simulink model "TST_DReqSwt_DD"  (R2016b)
settings: Solver=FixedStepDiscrete  StartTime=0.0  StopTime=simTime  FixedStep=sampleTime  RelTol=1e-3
values from neighbouring files (symbols this model uses):
  testCase = 1    [initTST_DReqSwt_DD_001.m]
libraries: simulink x4, UnitTest_Lib x2
settings Model: Creator=xinchangran  LastModifiedBy=xinchangran
settings DebuggingCC: SignalRangeChecking=error

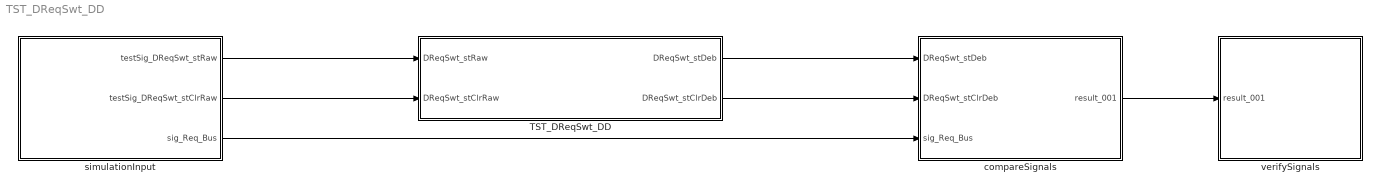
== system TST_DReqSwt_DD ==
  TST_DReqSwt_DD : Subsystem
  compareSignals : Subsystem
  simulationInput : Subsystem
  verifySignals : Subsystem
  wires:
  simulationInput/1(testSig_DReqSwt_stRaw) -> TST_DReqSwt_DD/1(DReqSwt_stRaw)
  simulationInput/2(testSig_DReqSwt_stClrRaw) -> TST_DReqSwt_DD/2(DReqSwt_stClrRaw)
  TST_DReqSwt_DD/1(DReqSwt_stDeb) -> compareSignals/1(DReqSwt_stDeb)
  TST_DReqSwt_DD/2(DReqSwt_stClrDeb) -> compareSignals/2(DReqSwt_stClrDeb)
  simulationInput/3(sig_Req_Bus) -> compareSignals/3(sig_Req_Bus)
  compareSignals/1(result_001) -> verifySignals/1(result_001)

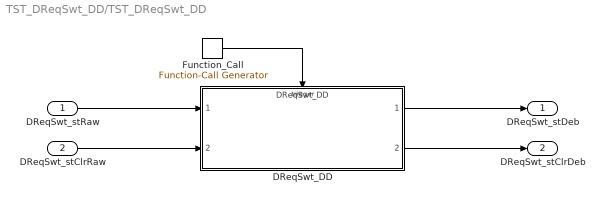
== system TST_DReqSwt_DD/TST_DReqSwt_DD ==
  DReqSwt_stRaw : Inport
  DReqSwt_stClrRaw : Inport  Port=2
  DReqSwt_DD : ModelReference  ModelNameDialog=DReqSwt_DD  SimulationMode=Normal  ModelReferenceVersion=1.17  TriggerPortName=function  TriggerPortTriggerType=function-call  TriggerPortStatesWhenEnabling=held
  Function_Call : simulink/Ports & Subsystems/Function-Call Generator  sample_time=sampleTime  numberOfIterations=1
  DReqSwt_stDeb : Outport
  DReqSwt_stClrDeb : Outport  Port=2
  wires:
  Function_Call/1 -> DReqSwt_DD/Trigger
  DReqSwt_stRaw/1 -> DReqSwt_DD/1
  DReqSwt_stClrRaw/1 -> DReqSwt_DD/2
  DReqSwt_DD/1 -> DReqSwt_stDeb/1
  DReqSwt_DD/2 -> DReqSwt_stClrDeb/1

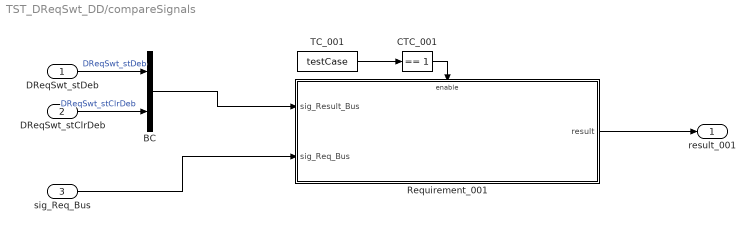
== system TST_DReqSwt_DD/compareSignals ==
  DReqSwt_stDeb : Inport
  DReqSwt_stClrDeb : Inport  Port=2
  sig_Req_Bus : Inport  Port=3
  BC : BusCreator  Inputs=2
  CTC_001 : simulink/Logic and Bit Operations/Compare To Constant  relop===  const=1  OutDataTypeStr=boolean
  Requirement_001 : Subsystem
  TC_001 : Constant  Value=testCase
  result_001 : Outport
  wires:
  DReqSwt_stDeb/1 -> BC/1  "DReqSwt_stDeb"
  DReqSwt_stClrDeb/1 -> BC/2  "DReqSwt_stClrDeb"
  TC_001/1 -> CTC_001/1
  CTC_001/1 -> Requirement_001/Enable
  sig_Req_Bus/1 -> Requirement_001/2(sig_Req_Bus)
  BC/1 -> Requirement_001/1(sig_Result_Bus)
  Requirement_001/1(result) -> result_001/1

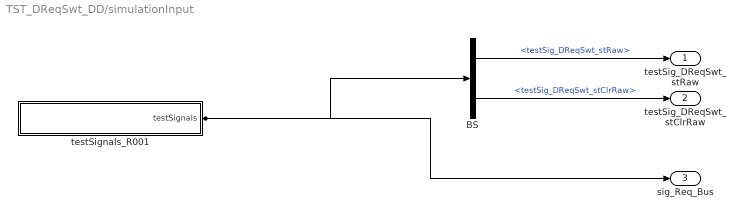
== system TST_DReqSwt_DD/simulationInput ==
  BS : BusSelector  OutputSignals=testSig_DReqSwt_stRaw,testSig_DReqSwt_stClrRaw
  testSignals_R001 : Subsystem
  testSig_DReqSwt_stRaw : Outport
  testSig_DReqSwt_stClrRaw : Outport  Port=2
  sig_Req_Bus : Outport  Port=3
  wires:
  BS/1 -> testSig_DReqSwt_stRaw/1  "<testSig_DReqSwt_stRaw>"
  BS/2 -> testSig_DReqSwt_stClrRaw/1  "<testSig_DReqSwt_stClrRaw>"
  testSignals_R001/1(testSignals) -> BS/1, sig_Req_Bus/1

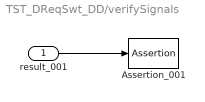
== system TST_DReqSwt_DD/verifySignals ==
  result_001 : Inport
  Assertion_001 : Assertion  Enabled=off
  wires:
  result_001/1 -> Assertion_001/1

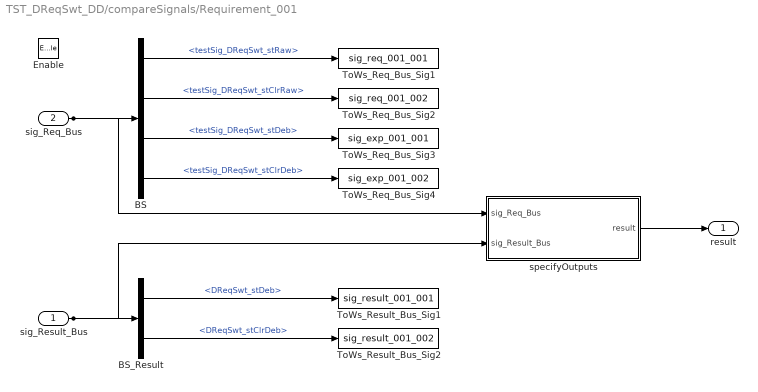
== system TST_DReqSwt_DD/compareSignals/Requirement_001 ==
  sig_Result_Bus : Inport
  sig_Req_Bus : Inport  Port=2
  Enable : EnablePort
  BS : BusSelector  OutputSignals=testSig_DReqSwt_stRaw,testSig_DReqSwt_stClrRaw,testSig_DReqSwt_stDeb,testSig_DReqSwt_stClrDeb
  BS_Result : BusSelector  OutputSignals=DReqSwt_stDeb,DReqSwt_stClrDeb
  ToWs_Req_Bus_Sig1 : ToWorkspace  VariableName=sig_req_001_001  SaveFormat=Structure With Time
  ToWs_Req_Bus_Sig2 : ToWorkspace  VariableName=sig_req_001_002  SaveFormat=Structure With Time
  ToWs_Req_Bus_Sig3 : ToWorkspace  VariableName=sig_exp_001_001  SaveFormat=Structure With Time
  ToWs_Req_Bus_Sig4 : ToWorkspace  VariableName=sig_exp_001_002  SaveFormat=Structure With Time
  ToWs_Result_Bus_Sig1 : ToWorkspace  VariableName=sig_result_001_001  SaveFormat=Structure With Time
  ToWs_Result_Bus_Sig2 : ToWorkspace  VariableName=sig_result_001_002  SaveFormat=Structure With Time
  specifyOutputs : Subsystem
  result : Outport
  wires:
  sig_Req_Bus/1 -> BS/1, specifyOutputs/1(sig_Req_Bus)
  BS/1 -> ToWs_Req_Bus_Sig1/1  "<testSig_DReqSwt_stRaw>"
  BS/2 -> ToWs_Req_Bus_Sig2/1  "<testSig_DReqSwt_stClrRaw>"
  BS/3 -> ToWs_Req_Bus_Sig3/1  "<testSig_DReqSwt_stDeb>"
  BS/4 -> ToWs_Req_Bus_Sig4/1  "<testSig_DReqSwt_stClrDeb>"
  sig_Result_Bus/1 -> BS_Result/1, specifyOutputs/2(sig_Result_Bus)
  BS_Result/1 -> ToWs_Result_Bus_Sig1/1  "<DReqSwt_stDeb>"
  BS_Result/2 -> ToWs_Result_Bus_Sig2/1  "<DReqSwt_stClrDeb>"
  specifyOutputs/1(result) -> result/1

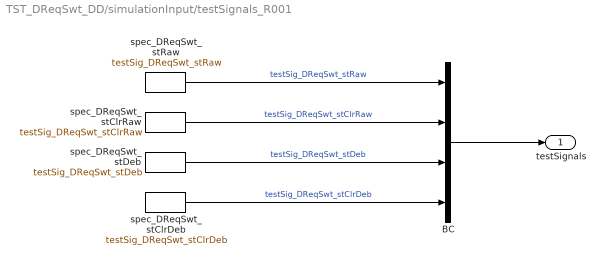
== system TST_DReqSwt_DD/simulationInput/testSignals_R001 ==
  BC : BusCreator  Inputs=4
  spec_DReqSwt_stClrDeb : FromWorkspace  VariableName=testSig_DReqSwt_stClrDeb  Interpolate=off  OutputAfterFinalValue=Holding final value
  spec_DReqSwt_stClrRaw : FromWorkspace  VariableName=testSig_DReqSwt_stClrRaw  Interpolate=off  OutputAfterFinalValue=Holding final value
  spec_DReqSwt_stDeb : FromWorkspace  VariableName=testSig_DReqSwt_stDeb  Interpolate=off  OutputAfterFinalValue=Holding final value
  spec_DReqSwt_stRaw : FromWorkspace  VariableName=testSig_DReqSwt_stRaw  Interpolate=off  OutputAfterFinalValue=Holding final value
  testSignals : Outport
  wires:
  BC/1 -> testSignals/1
  spec_DReqSwt_stRaw/1 -> BC/1  "testSig_DReqSwt_stRaw"
  spec_DReqSwt_stClrRaw/1 -> BC/2  "testSig_DReqSwt_stClrRaw"
  spec_DReqSwt_stDeb/1 -> BC/3  "testSig_DReqSwt_stDeb"
  spec_DReqSwt_stClrDeb/1 -> BC/4  "testSig_DReqSwt_stClrDeb"

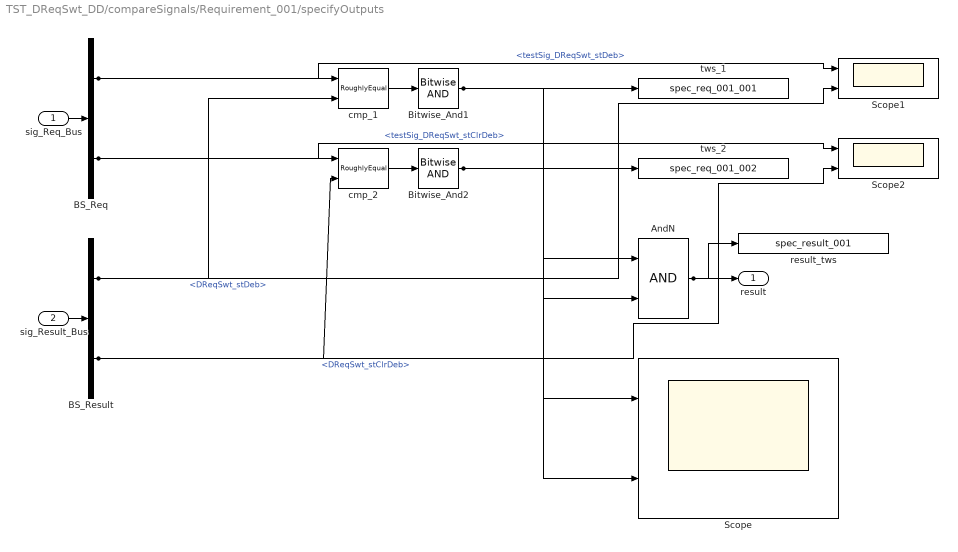
== system TST_DReqSwt_DD/compareSignals/Requirement_001/specifyOutputs ==
  sig_Req_Bus : Inport
  sig_Result_Bus : Inport  Port=2
  AndN : Logic
  BS_Req : BusSelector  OutputSignals=testSig_DReqSwt_stDeb,testSig_DReqSwt_stClrDeb
  BS_Result : BusSelector  OutputSignals=DReqSwt_stDeb,DReqSwt_stClrDeb
  Bitwise_And1 : simulink/Logic and Bit Operations/Bitwise Operator  logicop=AND  UseBitMask=off  BitMask=bin2dec('11011001')  BitMaskRealWorld=Stored Integer
  Bitwise_And2 : simulink/Logic and Bit Operations/Bitwise Operator  logicop=AND  UseBitMask=off  BitMask=bin2dec('11011001')  BitMaskRealWorld=Stored Integer
  Scope : Scope  NumInputPorts=2
  Scope1 : Scope  NumInputPorts=2
  Scope2 : Scope  NumInputPorts=2
  cmp_1 : UnitTest_Lib/RoughlyEqual  slope=0.1
  cmp_2 : UnitTest_Lib/RoughlyEqual  slope=0.1
  result_tws : ToWorkspace  VariableName=spec_result_001
  tws_1 : ToWorkspace  VariableName=spec_req_001_001
  tws_2 : ToWorkspace  VariableName=spec_req_001_002
  result : Outport
  wires:
  sig_Req_Bus/1 -> BS_Req/1
  sig_Result_Bus/1 -> BS_Result/1
  AndN/1 -> result/1, result_tws/1
  BS_Req/1 -> cmp_1/1, Scope1/1  "<testSig_DReqSwt_stDeb>"
  BS_Result/1 -> cmp_1/2, Scope1/2  "<DReqSwt_stDeb>"
  cmp_1/1 -> Bitwise_And1/1
  Bitwise_And1/1 -> tws_1/1, AndN/1, Scope/1
  BS_Req/2 -> cmp_2/1, Scope2/1  "<testSig_DReqSwt_stClrDeb>"
  BS_Result/2 -> cmp_2/2, Scope2/2  "<DReqSwt_stClrDeb>"
  cmp_2/1 -> Bitwise_And2/1
  Bitwise_And2/1 -> tws_2/1, AndN/2, Scope/2
